simulink model "Pcontrol"  (R2024b)
settings: Solver=VariableStepAuto  StartTime=0.0  StopTime=10.0  RelTol=1e-3
settings Model: Creator=fve2  LastModifiedBy=fve2

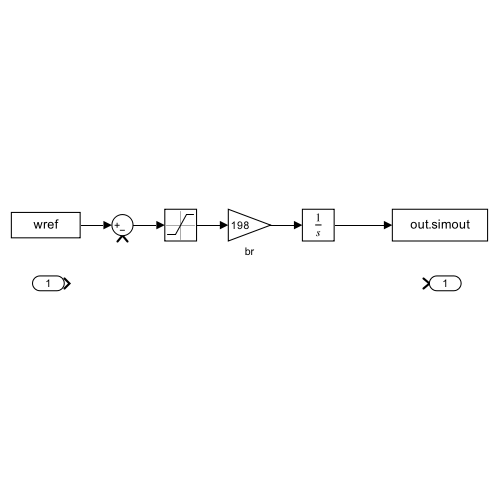
[thumbnail: Simulink's stored preview of the top-level diagram]
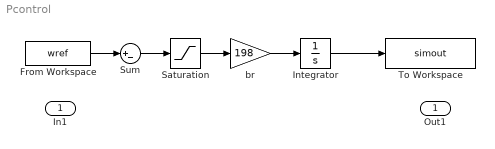
== system Pcontrol ==
  In1 : Inport
  From Workspace : FromWorkspace  VariableName=wref
  Integrator : Integrator
  Saturation : Saturate  UpperLimit=100  LowerLimit=0
  Sum : Sum  Inputs=|+-
  To Workspace : ToWorkspace  VariableName=simout  SaveFormat=Timeseries  SampleTime=-1
  br : Gain  Gain=198
  Out1 : Outport
  wires:
  Saturation/1 -> br/1
  br/1 -> Integrator/1
  From Workspace/1 -> Sum/1
  Sum/1 -> Saturation/1
  Integrator/1 -> To Workspace/1
